simulink model "Sistema"  (R2023a)
settings: Solver=ode1  StartTime=0.0  StopTime=0.1  FixedStep=1e-6  RelTol=1e-3
libraries: slpidlib x1
settings Model: Creator=apdy8  LastModifiedBy=apdy8
settings DataIOCC: ReturnWorkspaceOutputs=off  TimeSaveName=t
settings DebuggingCC: AlgebraicLoopMsg=none  ArtificialAlgebraicLoopMsg=none

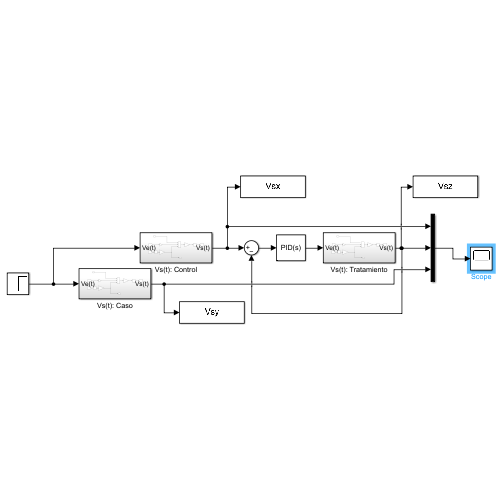
[thumbnail: Simulink's stored preview of the top-level diagram]
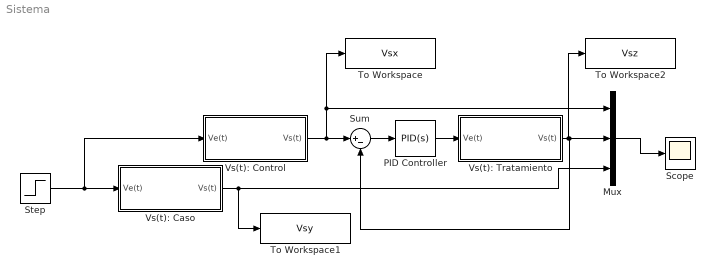
== system Sistema ==
  Mux : Mux  Inputs=3
  PID Controller : slpidlib/PID Controller  Controller=PID  Form=Parallel  TimeDomain=Continuous-time  UseExternalTs=off  SampleTime=-1  IntegratorMethod=Forward Euler  FilterMethod=Forward Euler  ControllerParametersSource=internal  P=14.2344066883988  I=12845.3383616807  UseKiTs=off  D=0.00371075715486635  N=1743057.57692824  UseFilter=on  TunerSelectOption=Transfer Function Based (PID Tuner App)  InitialConditionSource=internal  InitialConditionForIntegrator=0  InitialConditionForFilter=0  DifferentiatorICPrevScaledInput=0  ExternalReset=none  TrackingMode=off  Kt=1  LimitOutput=off  SatLimitsSource=internal  UpperSaturationLimit=inf  LowerSaturationLimit=-inf  LinearizeAsGain=on  AntiWindupMode=none  Kb=1  LimitIntegrator=off  UpperIntegratorSaturationLimit=inf  LowerIntegratorSaturationLimit=-inf  POutMin=[]  POutMax=[]  IOutMin=[]  IOutMax=[]  DOutMin=[]  DOutMax=[]  NOutMin=[]  NOutMax=[]  SumOutMin=[]  SumOutMax=[]  SaturationOutMin=[]  SaturationOutMax=[]  PParamMin=[]  PParamMax=[]  IParamMin=[]  IParamMax=[]  DParamMin=[]  DParamMax=[]  NParamMin=[]  NParamMax=[]  KbParamMin=[]  KbParamMax=[]  KtParamMin=[]  KtParamMax=[]  KbOutMin=[]  KbOutMax=[]  KtOutMin=[]  KtOutMax=[]  IntegratorOutMin=[]  IntegratorOutMax=[]  FilterOutMin=[]  FilterOutMax=[]  SumI1OutMin=[]  SumI1OutMax=[]  SumI2OutMin=[]  SumI2OutMax=[]  SumI3OutMin=[]  SumI3OutMax=[]  SumI4OutMin=[]  SumI4OutMax=[]  SumDOutMin=[]  SumDOutMax=[]  DifferentiatorOutMin=[]  DifferentiatorOutMax=[]  FilterDiffOutCoefMin=[]  FilterDiffOutCoefMax=[]  ReciprocalOutMin=[]  ReciprocalOutMax=[]  SumDenOutMin=[]  SumDenOutMax=[]  SumNumOutMin=[]  SumNumOutMax=[]  DivideOutMin=[]  DivideOutMax=[]  UdiffTsProdOutMin=[]  UdiffTsProdOutMax=[]  NTsProdOutMin=[]  NTsProdOutMax=[]  UintegralTsProdOutMin=[]  UintegralTsProdOutMax=[]  UngainTsProdOutMin=[]  UngainTsProdOutMax=[]  ClampingZeroOutDataTypeStr=Inherit: Inherit via back propagation  ClampingZeroOutMin=[]  ClampingZeroOutMax=[]  FilterDenConstantOutDataTypeStr=Inherit: Inherit via back propagation  FilterDenConstantOutMin=[]  FilterDenConstantOutMax=[]  PCopyOutDataTypeStr=Inherit: Inherit via back propagation  PCopyOutMin=[]  PCopyOutMax=[]  NCopyOutDataTypeStr=Inherit: Inherit via back propagation  NCopyOutMin=[]  NCopyOutMax=[]  IntegratorContinuousStateAttributes=''  IntegratorStateMustResolveToSignalObject=off  IntegratorRTWStateStorageClass=Auto  FilterContinuousStateAttributes=''  FilterStateMustResolveToSignalObject=off  FilterRTWStateStorageClass=Auto  ParallelPVariant=InternalParameters  IdealPVariant=Disabled  IVariant=InternalParameters  DVariant=InternalParameters  IntegratorVariant=Continuous  SatVariant=Disabled  AWVariant=Passthrough  PCopyVariant=Disabled  TRVariant=Disabled  FdbkBlocksVariant=Forward  IdealPFdbkVariant=Disabled  SatFdbkVariant=Disabled  DerivativeFilterVariant=ContFilter  NVariant=InternalParameters  NCopyVariant=Disabled  FilterICVariant=InternalICsFilter  IntegratorICVariant=InternalICs  ExternalResetVariant=Disabled  TRSumVariant=Passthrough  SumFdbkVariant=Disabled  SumVariant=Sum_PID  TsampFilterVariant=InternalTs  TsampNgainVariant=Passthrough  TsampIntegralVariant=Disabled_SignalSpec  ExternalSaturationOutDataTypeStr=Inherit: Same as second input
  Scope : Scope
  Step : Step  Time=0  SampleTime=0.001
  Sum : Sum  Inputs=|+-
  To Workspace : ToWorkspace  VariableName=Vsx  SampleTime=-1
  To Workspace1 : ToWorkspace  VariableName=Vsy  SampleTime=-1
  To Workspace2 : ToWorkspace  VariableName=Vsz  SampleTime=-1
  Vs(t): Caso : Subsystem
  Vs(t): Control : Subsystem
  Vs(t): Tratamiento : Subsystem
  wires:
  Mux/1 -> Scope/1
  Step/1 -> Vs(t): Control/1(Ve(t)), Vs(t): Caso/1(Ve(t))
  Vs(t): Control/1(Vs(t)) -> To Workspace/1, Mux/1, Sum/1
  Sum/1 -> PID Controller/1
  PID Controller/1 -> Vs(t): Tratamiento/1(Ve(t))
  Vs(t): Caso/1(Vs(t)) -> To Workspace1/1, Mux/3
  Vs(t): Tratamiento/1(Vs(t)) -> To Workspace2/1, Mux/2, Sum/2

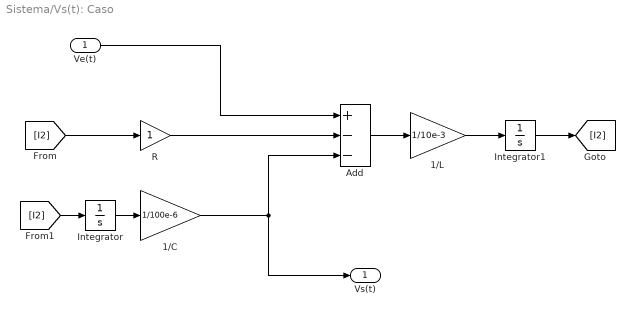
== system Sistema/Vs(t): Caso ==
  Ve(t) : Inport
  1/C : Gain  Gain=1/100e-6
  1/L : Gain  Gain=1/10e-3
  Add : Sum  Inputs=+--
  Integrator : Integrator
  Integrator1 : Integrator
  R : Gain
  Vs(t) : Outport
  wires:
  Ve(t)/1 -> Add/1
  [I2] -> R/1
  R/1 -> Add/2
  [I2] -> Integrator/1
  Integrator/1 -> 1/C/1
  1/C/1 -> Vs(t)/1, Add/3
  Add/1 -> 1/L/1
  1/L/1 -> Integrator1/1
  Integrator1/1 -> [I2]

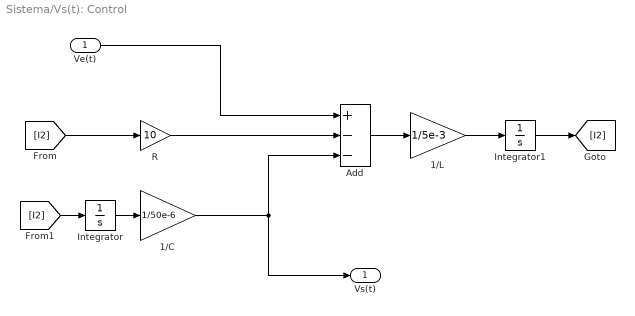
== system Sistema/Vs(t): Control ==
  Ve(t) : Inport
  1/C : Gain  Gain=1/50e-6
  1/L : Gain  Gain=1/5e-3
  Add : Sum  Inputs=+--
  Integrator : Integrator
  Integrator1 : Integrator
  R : Gain  Gain=10
  Vs(t) : Outport
  wires:
  Ve(t)/1 -> Add/1
  [I2] -> R/1
  R/1 -> Add/2
  [I2] -> Integrator/1
  Integrator/1 -> 1/C/1
  1/C/1 -> Vs(t)/1, Add/3
  Add/1 -> 1/L/1
  1/L/1 -> Integrator1/1
  Integrator1/1 -> [I2]

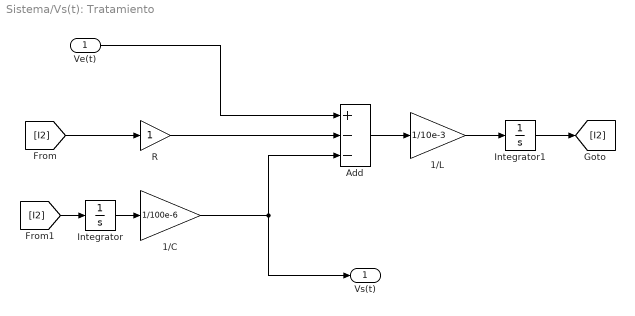
== system Sistema/Vs(t): Tratamiento ==
  Ve(t) : Inport
  1/C : Gain  Gain=1/100e-6
  1/L : Gain  Gain=1/10e-3
  Add : Sum  Inputs=+--
  Integrator : Integrator
  Integrator1 : Integrator
  R : Gain
  Vs(t) : Outport
  wires:
  Ve(t)/1 -> Add/1
  [I2] -> R/1
  R/1 -> Add/2
  [I2] -> Integrator/1
  Integrator/1 -> 1/C/1
  1/C/1 -> Vs(t)/1, Add/3
  Add/1 -> 1/L/1
  1/L/1 -> Integrator1/1
  Integrator1/1 -> [I2]
